simulink library "NeuroModelerLibrary"  (Simulink 10.2)
settings: Solver=ode45  StartTime=0.0  StopTime=10.0  RelTol=1e-3
libraries: $bdroot x672, simulink x5, neural x2
(part 1 of 5)
settings Model: Creator=Bakhshiev  LastModifiedBy=Bakhshiev

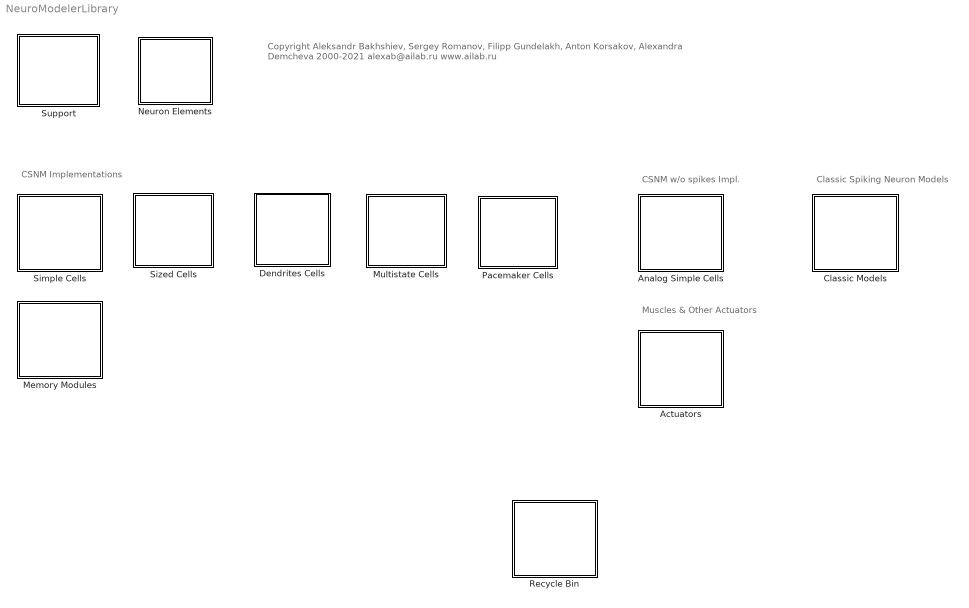
== system NeuroModelerLibrary ==
  note: CSNM Implementations
  note: Copyright Aleksandr Bakhshiev, Sergey Romanov, Filipp Gundelakh, Anton Korsakov, Alexandra Demcheva 2000-2021
      | alexab@ailab.ru
      | www.ailab.ru
  note: CSNM w/o spikes Impl.
  note: Muscles & Other Actuators
  note: Classic Spiking Neuron Models
  Actuators : Subsystem
  Analog Simple Cells : Subsystem
  Classic Models : Subsystem
  Dendrites Cells : Subsystem
  Memory Modules : Subsystem
  Multistate Cells : Subsystem
  Neuron Elements : Subsystem
  Pacemaker Cells : Subsystem
  Recycle Bin : Subsystem
  Simple Cells : Subsystem
  Sized Cells : Subsystem
  Support : Subsystem

== system NeuroModelerLibrary/Actuators ==
  Eye Muscle : Subsystem

== system NeuroModelerLibrary/Analog Simple Cells ==
  note: CSNM: version 0.2
  Simple Analog Neuron : Subsystem
  Simple Analog Neuron with PI : Subsystem  AncestorBlock=NeuroModelerLibrary/Analog Simple Cells/Simple Analog Neuron
  "Simple Tanh Analog Neuron " : Subsystem

== system NeuroModelerLibrary/Classic Models ==
  note: Neuron Models
  note: Synapse Models
  Alpha-Function Synapse (nonsmooth) : Subsystem  mask{tau_syn=2e-3, I_syn=1e-12, weight=1, delay=1e-3}
      mask prompts: tau_syn "Rise time of the exciatory synaptic alpha function"; I_syn "Synaptic current amplitude"
  Alpha-Function Synapse (smooth) : Subsystem  mask{tau_syn=2e-3, I_syn=1e-12, weight=1, delay=1e-3}
      mask prompts: tau_syn "Rise time of excitatory synaptic alpha function"; I_syn "Synaptic current amplitude"
  IaF Neuron : Subsystem  mask{tau_m=0.01, Cm=250e-12, I_const=0, E_L=-0.070, V_reset=-0.10, V_th=-0.055}
      mask prompts: tau_m "Membrane time constatnt"; Cm "Membrane capacity"; I_const "Constant input current"; E_L "Resting membrane potential"; V_reset "Reset membrane potential"; V_th "Threshold potential"
  IaF Neuron with refractory : Subsystem  mask{tau_m=0.01, Cm=250e-12, I_const=376e-12, E_L=-0.070, V_reset=-0.070, V_th=-0.055, tau_ref=0.002}
      mask prompts: tau_m "Membrane time constatnt"; Cm "Membrane capacity"; I_const "Constant input current"; E_L "Resting membrane potential"; V_reset "Reset membrane potential"; V_th "Threshold potential"; tau_ref "Refractory period"
  Static Synapse : Subsystem  mask{tau_syn=2e-3, I_syn=1e-8, weight=1, delay=1e-3}
      mask prompts: tau_syn "Rise time of the excitatory synaptic alpha function"; I_syn "Synaptic current amplitude"

== system NeuroModelerLibrary/Dendrites Cells ==
  note: CSNM: version 0.2
  Branching Dendrites Cell : Subsystem
  Branching Dendrites Cell ModGen : Subsystem  AncestorBlock=NeuroModelerLibrary/Dendrites Cells/Branching Dendrites Cell
  Branching Dendrites Cell ModGenSyn : Subsystem  AncestorBlock=NeuroModelerLibrary/Dendrites Cells/Branching Dendrites Cell
  Long Dendite Cell : Subsystem
  Long Dendite Cell ModGen : Subsystem  AncestorBlock=NeuroModelerLibrary/Dendrites Cells/Long Dendite Cell
  Long Dendite Cell ModGen(FBC) : Subsystem  AncestorBlock=NeuroModelerLibrary/Dendrites Cells/Long Dendite Cell
  Long Dendite Cell ModGenSyn : Subsystem  AncestorBlock=NeuroModelerLibrary/Dendrites Cells/Long Dendite Cell

== system NeuroModelerLibrary/Memory Modules ==
  note: CSNM: version 0.2
  Time-Memory Element : Subsystem
  Time-Memory PI Element : Subsystem

== system NeuroModelerLibrary/Multistate Cells ==
  note: CSNM: version 0.2
  Multistate Membrane Cell : Subsystem

== system NeuroModelerLibrary/Neuron Elements ==
  note: CSNM: version 0.1 (2010)
  note: CSNM: version 0.2 (2015)
  note: CSNM: version 0.3 (2021)
  CSNM Compartment : Subsystem  mask{ACm=1e-9, ARm=1e7, ECm=1e-9, ERm=1e7, ARFm=1e7, ERFm=1e7, U0=-0.070, sign=-1}
      mask prompts: ACm "Arresting Membrane Capacity"; ARm "Arresting Membrane Resistance"; ECm "Excitatory Membrane Capacity"; ERm "Excitatory Membrane Resistance"; ARFm "Feedback Arresting Resistance"; ERFm "Feedback Excitatory Resistance"; U0 "Synaptic EMF"; sign "Synaptic Weight Sign"
  CSNM LTZone : Subsystem  mask(Ion pump){NM=1, FB=2, T=-0.055, switchOff=-0.1}
      mask prompts: NM "Number of Input Membranes"; FB "Feedback Coeff"; T "On Threshold"; switchOff "Off Threshold"
  CSNM Synapse : Subsystem  mask{SecretionTC=0.001, DecompositionTC=0.005, UseKsi=off, Rs=2e7, ksi=1, U0=-0.070, Weight=1, sign=off}
      mask prompts: SecretionTC "Mediator Secretion"; DecompositionTC "Mediator Decomposition"; UseKsi "Use Presynaptic Inhubition"; Rs "Synaptic Resistance"; U0 "Synaptic EMF"; Weight "Synaptic Weight"; sign "Synaptic Weight Sign"
  CSNM Synapse-D : Subsystem  mask{SecretionTC=0.001, DecompositionTC=0.005, UseKsi=off, Rs=2e7, ksi=1, U0=-0.070, Weight=1, sign=off}
      mask prompts: SecretionTC "Mediator Secretion"; DecompositionTC "Mediator Decomposition"; UseKsi "Use Presynaptic Inhubition"; Rs "Synaptic Resistance"; U0 "Synaptic EMF"; Weight "Synaptic Weight"; sign "Synaptic Weight Sign"
  ContLTZone : Subsystem
  IaF Compartment : Subsystem  mask{tau_m=0.01, Cm=250e-12, I_const=0, E_L=-0.070, V_reset=-0.10, V_th=-0.055}
      mask prompts: tau_m "Membrane time constatnt"; Cm "Membrane capacity"; I_const "Constant input current"; E_L "Resting membrane potential"; V_reset "Reset membrane potential"; V_th "Threshold potential"
  IaF LTZone : Subsystem  mask{tau_m=0.01, Cm=250e-12, I_const=0, E_L=-0.070, V_reset=-0.10, V_th=-0.055}
      mask prompts: tau_m "Membrane time constatnt"; Cm "Membrane capacity"; I_const "Constant input current"; E_L "Resting membrane potential"; V_reset "Reset membrane potential"; V_th "Threshold potential"
  Ion System : Subsystem
  Ion System v0.1 : Subsystem
  LTZone : Subsystem  mask(Ion pump){NM=1, FB=1.7, IT=0.005, T=0.001}
      mask prompts: NM "Number of Input Membranes"; FB "Feedback Coeff"; IT "Input Time Constant"; T "Threshold"
  LTZone v0.1 : Subsystem  mask(Ion pump){Rc=1, Cc=0.001, RR=1, IT=0.005, T=10}
      mask prompts: Rc "Channel resistance"; Cc "Channel capacity"; RR "Recharge Resistance"; IT "Input TC"; T "Threshold"
  LTZoneV2 : Subsystem  mask(Ion pump){NM=1, FB=2, IT=0.001, T=-0.055, inertia=on, switchOff=-0.1}
      mask prompts: NM "Number of Input Membranes"; FB "Feedback Coeff"; IT "Input Time Constant"; T "Threshold"; inertia "Use inertia link"; switchOff "Switch off point"
  Multistate Membrane : Subsystem
  Neuro Membrane v0.1 : Subsystem  mask{ACm=0.1, ARm=0.1, ECm=0.01, ERm=0.1}
      mask prompts: ACm "Arresting Membrane Capacity"; ARm "Arresting Membrane Resistance"; ECm "Excitatory Membrane Capacity"; ERm "Excitatory Membrane Resistance"
  Simple Membrane : Subsystem  mask{ACm=1e-9, ARm=1e7, ECm=1e-9, ERm=1e7, ARFm=1e8, ERFm=1e8}
      mask prompts: ACm "Arresting Membrane Capacity"; ARm "Arresting Membrane Resistance"; ECm "Excitatory Membrane Capacity"; ERm "Excitatory Membrane Resistance"; ARFm "Feedback Arresting Resistance"; ERFm "Feedback Excitatory Resistance"
  Simple Synapse : $bdroot/Neuron Elements/Synapse  SecretionTC=0.001  DecompositionTC=0.01  UseKsi=off  ksi=2  gamma=1e8
  Synapse : Subsystem  mask{SecretionTC=0.001, DecompositionTC=0.01, UseKsi=on, ksi=2, gamma=1e8}
      mask prompts: SecretionTC "Mediator Secretion"; DecompositionTC "Mediator Decomposition"; UseKsi "Use Presynaptic Inhubition"
  Synapse Ion System v0.1 : Subsystem
  Synapse Membrane v0.1 : Subsystem  mask{ACm=0.1, ARm=0.1, ECm=0.01, ERm=0.1}
      mask prompts: ACm "Arresting Membrane Capacity"; ARm "Arresting Membrane Resistance"; ECm "Excitatory Membrane Capacity"; ERm "Excitatory Membrane Resistance"
  Synapse PresynInh v0.1 : $bdroot/Neuron Elements/Synapse v0.1  SecretionTC=0.001  DecompositionTC=0.1  ksi=2  gamma=1
  Synapse v0.1 : Subsystem  mask{SecretionTC=0.001, DecompositionTC=0.1, ksi=1, gamma=1}
      mask prompts: SecretionTC "Mediator Secretion"; DecompositionTC "Mediator Decomposition"

== system NeuroModelerLibrary/Pacemaker Cells ==
  note: CSNM: version 0.2
  Pacemaker1-1 Cell : Subsystem
  Pacemaker1-2 Cell : Subsystem
  Pacemaker1-3 Cell : Subsystem
  Pacemaker1-4 Cell : Subsystem
  Pacemaker2 Cell : Subsystem
  Pacemaker3 Cell : Subsystem
  Pacemaker4 Cell : Subsystem
  Pacemaker4x4 Cell : Subsystem
  Slow Pacemaker Cell : Subsystem

== system NeuroModelerLibrary/Recycle Bin ==
  note: Neural Networks Samples
  note: Neuron Samples
  note: Neuron Parts Samples
  Dendrite Neuron  Samples : Subsystem
  Membrane Samples : Subsystem
  Multistate Neuron  Samples : Subsystem
  PCN1 : Subsystem
  PCN2 : Subsystem
  Pacemaker Samples : Subsystem
  RCN : Subsystem
  Simple  Neural Networks : Subsystem
  Simple Neuron Samples : Subsystem
  Size Neuron  Samples : Subsystem
  Synapse Samples : Subsystem
  TCN : Subsystem

== system NeuroModelerLibrary/Simple Cells ==
  note: CSNM: version 0.2
  note: CSNM: version 0.1
  Afferent1 : Subsystem  mask{ExpCoeff=0.001, IncCoeff=0.999}
      mask prompts: ExpCoeff "Input Exp Coeff"; IncCoeff "Input Inc Coeff"
      mask DialogControl AffParams Prompt: Afferent Parameters
  Electric Simple Cell : Subsystem
  Electric Simple2 Cell : Subsystem
  Large  NewNeuron v0.1 : Subsystem
  Large PresynInh  NewNeuron v0.1 : Subsystem  AncestorBlock="NeuroModelerLibrary/Simple Cells/Large  NewNeuron v0.1"
  Simple Cell : Subsystem
  Simple Cell - Inertial : Subsystem  AncestorBlock=NeuroModelerLibrary/Simple Cells/Simple Cell
  Simple Cell MembraneCap : Subsystem
  Simple Cell MembraneCap[2] : Subsystem
  Small  NewNeuron v0.1 : Subsystem
  Small PresynInh NewNeuron v0.1 : Subsystem  AncestorBlock="NeuroModelerLibrary/Simple Cells/Small  NewNeuron v0.1"

== system NeuroModelerLibrary/Sized Cells ==
  note: CSNM: version 0.2
  note: CSNM: version 0.3
  note: Segmented IaF
  CSNM1x0 : Subsystem
  CSNM1x1 : Subsystem
  CSNM1x2 : Subsystem
  CSNM1x3 : Subsystem
  CSNM1x4-Syn4 : Subsystem
  CSNM2x0 : Subsystem
  CSNM2x1 : Subsystem
  CSNM2x2 : Subsystem
  CSNM2x3 : Subsystem
  CSNM3x0 : Subsystem
  CSNM3x1 : Subsystem
  CSNM3x2 : Subsystem
  CSNM3x3 : Subsystem
  CSNM4x0 : Subsystem
  CSNM4x1 : Subsystem
  CSNM4x2 : Subsystem
  CSNM4x3 : Subsystem
  Cell IaF 1x4 : Subsystem
  Cell IaF 1x4-Syn4 : Subsystem
  Cell IaF 2x4 : Subsystem
  Cell IaF 3x4 : Subsystem
  Cell IaF 4x4 : Subsystem
  Size Cell : Subsystem
  Size2 Cell : Subsystem
  Size3 Cell : Subsystem
  Size3 Cell ModSynS1A1 : Subsystem
  Size4 Cell : Subsystem
  Size6 Cell : Subsystem

== system NeuroModelerLibrary/Support ==
  Electric Engine Model : Subsystem
  Inertial Link : Subsystem
  Inertial Link With Reset : Subsystem
  Sign Separator : Subsystem
  Two-output Pulse Generator : Subsystem  mask{A=1, P1=200, P2=200, PW=1, ST=0.001, OOn1=0.5, OOff1=0.6, OOn2=1.1, OOff2=1.2}
      mask prompts: A "Amplitude"; P1 "Out1: Period (number of samples)"; P2 "Out2: Period (number of samples)"; PW "Pulse Width (number of samples)"; ST "Sample Time"; OOn1 "Out1 On (seconds)"; OOff1 "Out1 Off (seconds)"; OOn2 "Out2 On (seconds)"; OOff2 "Out2 Off (seconds)"

== system NeuroModelerLibrary/Actuators/Eye Muscle ==
  In1 : Inport
  Gain : Gain  Gain=380
  Gain1 : Gain  Gain=0.75
  Gain2 : Gain  Gain=195
  Gain3 : Gain  Gain=0.75
  Gain4 : Gain  Gain=30
  Gain5 : Gain  Gain=0.45
  Integrator : Integrator
  Integrator1 : Integrator
  Integrator2 : Integrator
  Subtract : Sum  Inputs=+--
  Subtract1 : Sum  Inputs=+-
  Out1 : Outport
  wires:
  In1/1 -> Subtract/1
  Subtract/1 -> Gain/1
  Gain1/1 -> Subtract/3
  Integrator/1 -> Gain1/1, Subtract1/1
  Integrator1/1 -> Gain4/1, Gain3/1
  Gain2/1 -> Integrator1/1
  Gain4/1 -> Integrator2/1
  Subtract1/1 -> Gain2/1
  Gain/1 -> Integrator/1
  Integrator2/1 -> Out1/1, Gain5/1
  Gain3/1 -> Subtract1/2
  Gain5/1 -> Subtract/2

== system NeuroModelerLibrary/Analog Simple Cells/Simple Analog Neuron ==
  Ex Input 1 : Inport
  Ex Input 2 : Inport  Port=2
  Ar Input 2 : Inport  Port=3
  Ar Input 1 : Inport  Port=4
  C2 : Constant
  C3 : Constant  Value=-1
  ContLTZone1 : $bdroot/Neuron Elements/ContLTZone  SystemSampleTime=-1  VariantActivationTime=update diagram  Latency=0  AutoFrameSizeCalculation=off
  Simple Membrane1 : $bdroot/Neuron Elements/Simple Membrane  ACm=1e-9  ARm=1e7  ECm=1e-9  ERm=1e7  ARFm=1e8  ERFm=1e8
  Simple Synapse{,1..3} (4 alike) : $bdroot/Neuron Elements/Synapse  SecretionTC=0.001  DecompositionTC=0.01  UseKsi=off  ksi=2  gamma=1e8
  Sum4 : Sum  InputSameDT=on  SaturateOnIntegerOverflow=on  OutDataTypeStr=Inherit: Same as first input
  Sum7 : Sum  InputSameDT=on  SaturateOnIntegerOverflow=on  OutDataTypeStr=Inherit: Same as first input
  Sum8 : Sum  InputSameDT=on  SaturateOnIntegerOverflow=on  OutDataTypeStr=Inherit: Same as first input
  Out : Outport  VectorParamsAs1DForOutWhenUnconnected=off
  Potential : Outport  Port=2  VectorParamsAs1DForOutWhenUnconnected=off
  wires:
  Ex Input 2/1 -> Simple Synapse1/1
  ContLTZone1/1 -> Out/1
  Simple Synapse3/1 -> Sum8/2
  Simple Synapse2/1 -> Sum8/1
  Sum8/1 -> Simple Membrane1/5
  Ar Input 2/1 -> Simple Synapse3/1
  Simple Synapse1/1 -> Sum4/2
  Simple Synapse/1 -> Sum4/1
  Sum4/1 -> Simple Membrane1/1
  Ar Input 1/1 -> Simple Synapse2/1
  Ex Input 1/1 -> Simple Synapse/1
  Sum7/1 -> ContLTZone1/1, Potential/1
  Simple Membrane1/2 -> Sum7/2
  Simple Membrane1/1 -> Sum7/1
  C3/1 -> Simple Membrane1/4
  C2/1 -> Simple Membrane1/2

== system NeuroModelerLibrary/Analog Simple Cells/Simple Analog Neuron with PI ==
  Ex Input 1 : Inport
  Ex Input 2 : Inport  Port=2
  Ar Input 2 : Inport  Port=3
  Ar Input 1 : Inport  Port=4
  C2 : Constant
  C3 : Constant  Value=-1
  ContLTZone1 : $bdroot/Neuron Elements/ContLTZone  SystemSampleTime=-1  VariantActivationTime=update diagram  Latency=0  AutoFrameSizeCalculation=off
  Simple Membrane1 : $bdroot/Neuron Elements/Simple Membrane  ACm=1e-9  ARm=1e7  ECm=1e-9  ERm=1e7  ARFm=1e8  ERFm=1e8
  Simple Synapse{,1..3} (4 alike) : $bdroot/Neuron Elements/Synapse  SecretionTC=0.001  DecompositionTC=0.01  UseKsi=on  ksi=2  gamma=1e8
  Sum4 : Sum  InputSameDT=on  SaturateOnIntegerOverflow=on  OutDataTypeStr=Inherit: Same as first input
  Sum7 : Sum  InputSameDT=on  SaturateOnIntegerOverflow=on  OutDataTypeStr=Inherit: Same as first input
  Sum8 : Sum  InputSameDT=on  SaturateOnIntegerOverflow=on  OutDataTypeStr=Inherit: Same as first input
  Out : Outport  VectorParamsAs1DForOutWhenUnconnected=off
  Potential : Outport  Port=2  VectorParamsAs1DForOutWhenUnconnected=off
  wires:
  Ex Input 2/1 -> Simple Synapse1/1
  ContLTZone1/1 -> Out/1
  Simple Synapse3/1 -> Sum8/2
  Simple Synapse2/1 -> Sum8/1
  Sum8/1 -> Simple Membrane1/5
  Ar Input 2/1 -> Simple Synapse3/1
  Simple Synapse1/1 -> Sum4/2
  Simple Synapse/1 -> Sum4/1
  Sum4/1 -> Simple Membrane1/1
  Ar Input 1/1 -> Simple Synapse2/1
  Ex Input 1/1 -> Simple Synapse/1
  Sum7/1 -> ContLTZone1/1, Potential/1
  Simple Membrane1/2 -> Sum7/2
  Simple Membrane1/1 -> Sum7/1
  C3/1 -> Simple Membrane1/4
  C2/1 -> Simple Membrane1/2

== system NeuroModelerLibrary/Analog Simple Cells/Simple Tanh Analog Neuron  ==
  Ex Input 1 : Inport
  Ex Input 2 : Inport  Port=2
  Ar Input 2 : Inport  Port=3
  Ar Input 1 : Inport  Port=4
  C2 : Constant
  C3 : Constant  Value=-1
  Simple Membrane1 : $bdroot/Neuron Elements/Simple Membrane  ACm=1e-9  ARm=1e7  ECm=1e-9  ERm=1e7  ARFm=1e8  ERFm=1e8
  Simple Synapse{,1..3} (4 alike) : $bdroot/Neuron Elements/Simple Synapse  SecretionTC=0.001  DecompositionTC=0.01  gamma=1e8
  Sum4 : Sum  InputSameDT=on  SaturateOnIntegerOverflow=on  OutDataTypeStr=Inherit: Same as first input
  Sum7 : Sum  InputSameDT=on  SaturateOnIntegerOverflow=on  OutDataTypeStr=Inherit: Same as first input
  Sum8 : Sum  InputSameDT=on  SaturateOnIntegerOverflow=on  OutDataTypeStr=Inherit: Same as first input
  tansig : neural/Transfer Functions/tansig
  Out : Outport  VectorParamsAs1DForOutWhenUnconnected=off
  Potential : Outport  Port=2  VectorParamsAs1DForOutWhenUnconnected=off
  wires:
  C2/1 -> Simple Membrane1/2
  C3/1 -> Simple Membrane1/4
  Simple Membrane1/1 -> Sum7/1
  Simple Membrane1/2 -> Sum7/2
  Sum7/1 -> tansig/1, Potential/1
  Ex Input 1/1 -> Simple Synapse/1
  Ar Input 1/1 -> Simple Synapse2/1
  Sum4/1 -> Simple Membrane1/1
  Simple Synapse/1 -> Sum4/1
  Simple Synapse1/1 -> Sum4/2
  Ar Input 2/1 -> Simple Synapse3/1
  Sum8/1 -> Simple Membrane1/5
  Simple Synapse2/1 -> Sum8/1
  Simple Synapse3/1 -> Sum8/2
  tansig/1 -> Out/1
  Ex Input 2/1 -> Simple Synapse1/1

== system NeuroModelerLibrary/Classic Models/Alpha-Function Synapse (nonsmooth) ==
  pulse input : Inport
  -1/tau_syn : Gain  Gain=-1/(tau_syn)
  Clock : Clock
  Constant : Constant
  Constant1 : Constant  Value=0
  Constant2 : Constant  Value=0
  Delay : TransportDelay  DelayTime=delay
  I_syn : Gain  Gain=I_syn
  Math Function : Math  SaturateOnIntegerOverflow=on
  MinMax Running Resettable : simulink/Math Operations/MinMax Running Resettable  Function=max  vinit=0.0
  Product1 : Product
  Sum : Sum  Inputs=-+|
  Switch : Switch  Criteria=u2 > Threshold
  Switch1 : Switch  Criteria=u2 > Threshold
  Triggered Subsystem : Subsystem  TreatAsAtomicUnit=on
  Weight : Gain  Gain=weight
  i_syn : Outport
  wires:
  Delay/1 -> i_syn/1
  Switch1/1 -> Weight/1
  MinMax Running Resettable/1 -> Switch1/2
  Product1/1 -> Switch1/1
  Constant2/1 -> Switch1/3
  Constant/1 -> Switch/1
  Constant1/1 -> Switch/3
  Triggered Subsystem/1(Out1) -> Sum/1
  pulse input/1 -> MinMax Running Resettable/1, Triggered Subsystem/Trigger
  Clock/1 -> Triggered Subsystem/1(In1), Sum/2
  Switch/1 -> Product1/2
  Math Function/1 -> I_syn/1
  -1/tau_syn/1 -> Math Function/1
  Sum/1 -> Switch/2, -1/tau_syn/1
  Weight/1 -> Delay/1
  I_syn/1 -> Product1/1

== system NeuroModelerLibrary/Classic Models/Alpha-Function Synapse (smooth) ==
  pulse input : Inport
  -1/tau_syn : Gain  Gain=-1/(tau_syn)
  1/tau_syn : Gain  Gain=1/(tau_syn)
  Clock : Clock
  Constant : Constant
  Constant1 : Constant  Value=0
  Constant2 : Constant  Value=0
  Delay : TransportDelay  DelayTime=delay
  Gain4 : Gain  Gain=exp(1)
  I_syn : Gain  Gain=I_syn
  Math Function : Math  SaturateOnIntegerOverflow=on
  MinMax Running Resettable : simulink/Math Operations/MinMax Running Resettable  Function=max  vinit=0.0
  Product : Product
  Product1 : Product
  Sum : Sum  Inputs=-+|
  Switch : Switch  Criteria=u2 > Threshold
  Switch1 : Switch  Criteria=u2 > Threshold
  Triggered Subsystem : Subsystem  TreatAsAtomicUnit=on
  Weight : Gain  Gain=weight
  i_syn : Outport
  wires:
  Delay/1 -> i_syn/1
  Switch1/1 -> Weight/1
  MinMax Running Resettable/1 -> Switch1/2
  Product1/1 -> Switch1/1
  Constant2/1 -> Switch1/3
  Product/1 -> I_syn/1
  Constant/1 -> Switch/1
  Constant1/1 -> Switch/3
  Triggered Subsystem/1(Out1) -> Sum/1
  pulse input/1 -> MinMax Running Resettable/1, Triggered Subsystem/Trigger
  Clock/1 -> Triggered Subsystem/1(In1), Sum/2
  Switch/1 -> Product1/2
  Math Function/1 -> Product/2
  -1/tau_syn/1 -> Math Function/1
  Gain4/1 -> 1/tau_syn/1
  Sum/1 -> Gain4/1, -1/tau_syn/1, Switch/2
  Weight/1 -> Delay/1
  1/tau_syn/1 -> Product/1
  I_syn/1 -> Product1/1

== system NeuroModelerLibrary/Classic Models/IaF Neuron ==
  i_syn : Inport
  Constant1 : Constant  Value=V_reset
  Constant10 : Constant  Value=tau_m
  Constant11 : Constant  Value=E_L
  Constant12 : Constant  Value=I_const
  Constant2 : Constant
  Constant6 : Constant  Value=0
  Gain1 : Gain
  Gain2 : Gain  Gain=tau_m/Cm
  Gain3 : Gain  Gain=tau_m/Cm
  Inertial Link With Reset : $bdroot/Support/Inertial Link With Reset  SystemSampleTime=-1  VariantActivationTime=update diagram  Latency=0  AutoFrameSizeCalculation=off
  S1 : Switch  Threshold=V_th  SaturateOnIntegerOverflow=on  InputSameDT=on
  S3 : Switch  Threshold=V_th  SaturateOnIntegerOverflow=on  InputSameDT=on
  Sum1 : Sum
  Sum3 : Sum
  Vm : Outport
  wires:
  S3/1 -> Vm/1
  i_syn/1 -> Gain3/1
  S1/1 -> Inertial Link With Reset/4
  Constant1/1 -> Inertial Link With Reset/3, S3/1
  Inertial Link With Reset/1 -> S3/2, S3/3, S1/2
  Gain1/1 -> Inertial Link With Reset/1
  Sum3/1 -> Gain1/1
  Constant6/1 -> S1/3
  Constant2/1 -> S1/1
  Gain2/1 -> Sum1/2
  Sum1/1 -> Sum3/1
  Gain3/1 -> Sum1/1
  Constant10/1 -> Inertial Link With Reset/2
  Constant11/1 -> Sum3/2
  Constant12/1 -> Gain2/1

== system NeuroModelerLibrary/Classic Models/IaF Neuron with refractory ==
  i_syn : Inport
  Clock : Clock
  Constant1 : Constant  Value=V_reset
  Constant10 : Constant  Value=tau_m
  Constant11 : Constant  Value=E_L
  Constant12 : Constant  Value=I_const
  Constant2 : Constant
  Constant3 : Constant  Value=E_L
  Constant4 : Constant
  Constant5 : Constant  Value=0
  Constant6 : Constant  Value=0
  Gain3 : Gain  Gain=tau_m/Cm
  Inertial Link With Reset1 : $bdroot/Support/Inertial Link With Reset  SystemSampleTime=-1  VariantActivationTime=update diagram  Latency=0  AutoFrameSizeCalculation=off
  S1 : Switch  Threshold=V_th  SaturateOnIntegerOverflow=on  InputSameDT=on
  S2 : Switch  Threshold=tau_ref  SaturateOnIntegerOverflow=on  InputSameDT=on
  S3 : Switch  Threshold=V_th  SaturateOnIntegerOverflow=on  InputSameDT=on
  S4 : Switch  Threshold=V_th - 0.000005  SaturateOnIntegerOverflow=on  InputSameDT=on
  Sum : Sum  Inputs=-+|
  Sum1 : Sum
  Sum3 : Sum
  Triggered Subsystem : Subsystem  TreatAsAtomicUnit=on
  Vm : Outport
  wires:
  S4/1 -> Triggered Subsystem/Trigger
  Constant5/1 -> S4/3
  Inertial Link With Reset1/1 -> S1/2, S3/2, S3/3, S4/2
  Constant4/1 -> S4/1
  Constant3/1 -> S2/3
  S2/1 -> Vm/1
  Sum/1 -> S2/2
  Clock/1 -> Triggered Subsystem/1(In1), Sum/2
  Triggered Subsystem/1(Out1) -> Sum/1
  Gain3/1 -> Sum3/1  "Input"
  S3/1 -> S2/1
  S1/1 -> Inertial Link With Reset1/4
  Constant1/1 -> Inertial Link With Reset1/3, S3/1
  Sum3/1 -> Inertial Link With Reset1/1  "Value"
  Constant6/1 -> S1/3
  Constant2/1 -> S1/1
  Constant12/1 -> Sum1/2
  Sum1/1 -> Gain3/1
  i_syn/1 -> Sum1/1
  Constant10/1 -> Inertial Link With Reset1/2
  Constant11/1 -> Sum3/2

== system NeuroModelerLibrary/Classic Models/Static Synapse ==
  pulse input : Inport
  Gain : Gain  Gain=weight
  Gain6 : Gain  Gain=I_syn
  Transfer Fcn : TransferFcn  Denominator="[(tau_syn*tau_syn)  (2*tau_syn)  1]"
  Transport Delay : TransportDelay  DelayTime=delay
  i_syn : Outport
  wires:
  pulse input/1 -> Transfer Fcn/1
  Transfer Fcn/1 -> Gain6/1
  Gain6/1 -> Gain/1
  Gain/1 -> Transport Delay/1
  Transport Delay/1 -> i_syn/1

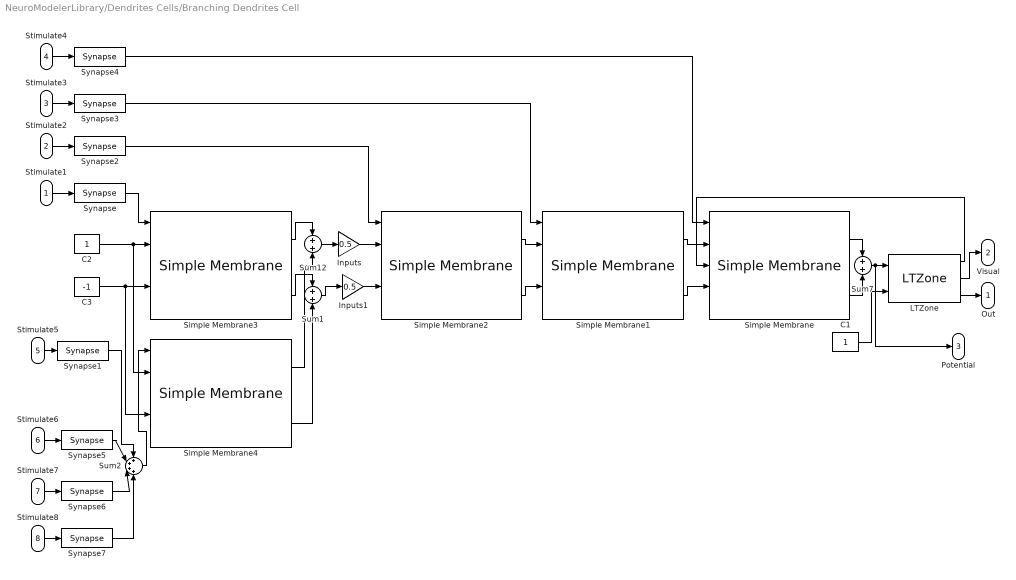
== system NeuroModelerLibrary/Dendrites Cells/Branching Dendrites Cell ==
  Stimulate1 : Inport
  Stimulate2 : Inport  Port=2
  Stimulate3 : Inport  Port=3
  Stimulate4 : Inport  Port=4
  Stimulate5 : Inport  Port=5
  Stimulate6 : Inport  Port=6
  Stimulate7 : Inport  Port=7
  Stimulate8 : Inport  Port=8
  C1 : Constant
  C2 : Constant
  C3 : Constant  Value=-1
  Inputs : Gain  Gain=0.5  OutDataTypeStr=Inherit: Same as input  ParamDataTypeStr=Inherit: Same as input
  Inputs1 : Gain  Gain=0.5  OutDataTypeStr=Inherit: Same as input  ParamDataTypeStr=Inherit: Same as input
  LTZone : $bdroot/Neuron Elements/LTZone  NM=1  FB=1.7  IT=0.005  T=0.001
  Simple Membrane{,1..4} (5 alike) : $bdroot/Neuron Elements/Simple Membrane  ACm=1e-9  ARm=1e7  ECm=1e-9  ERm=1e7  ARFm=1e8  ERFm=1e8
  Sum1 : Sum  InputSameDT=on  SaturateOnIntegerOverflow=on  OutDataTypeStr=Inherit: Same as first input
  Sum12 : Sum  InputSameDT=on  SaturateOnIntegerOverflow=on  OutDataTypeStr=Inherit: Same as first input
  Sum2 : Sum  Inputs=++++  InputSameDT=on  SaturateOnIntegerOverflow=on  OutDataTypeStr=Inherit: Same as first input
  Sum7 : Sum  InputSameDT=on  SaturateOnIntegerOverflow=on  OutDataTypeStr=Inherit: Same as first input
  Synapse{,1..7} (8 alike) : $bdroot/Neuron Elements/Synapse  SecretionTC=0.001  DecompositionTC=0.01  UseKsi=on  ksi=2  gamma=1e8
  Out : Outport  VectorParamsAs1DForOutWhenUnconnected=off
  Visual : Outport  Port=2  VectorParamsAs1DForOutWhenUnconnected=off
  Potential : Outport  Port=3  VectorParamsAs1DForOutWhenUnconnected=off
  wires:
  Synapse7/1 -> Sum2/4
  Stimulate8/1 -> Synapse7/1
  Synapse6/1 -> Sum2/3
  Stimulate7/1 -> Synapse6/1
  Stimulate6/1 -> Synapse5/1
  Stimulate4/1 -> Synapse4/1
  Synapse4/1 -> Simple Membrane/1
  Stimulate3/1 -> Synapse3/1
  Synapse3/1 -> Simple Membrane1/1
  Stimulate2/1 -> Synapse2/1
  Synapse2/1 -> Simple Membrane2/1
  Synapse/1 -> Simple Membrane3/1
  C2/1 -> Simple Membrane4/2, Simple Membrane3/2
  C3/1 -> Simple Membrane4/4, Simple Membrane3/4
  LTZone/2 -> Visual/1
  LTZone/3 -> Out/1
  C1/1 -> LTZone/2
  Stimulate1/1 -> Synapse/1
  Stimulate5/1 -> Synapse1/1
  Simple Membrane1/1 -> Simple Membrane/2
  Simple Membrane1/2 -> Simple Membrane/4
  Sum7/1 -> Potential/1, LTZone/1
  LTZone/1 -> Simple Membrane/3
  Simple Membrane/1 -> Sum7/1
  Simple Membrane/2 -> Sum7/2
  Simple Membrane4/2 -> Sum1/2
  Simple Membrane4/1 -> Sum12/2
  Sum12/1 -> Inputs/1
  Sum1/1 -> Inputs1/1
  Simple Membrane3/2 -> Sum1/1
  Simple Membrane3/1 -> Sum12/1
  Simple Membrane2/1 -> Simple Membrane1/2
  Simple Membrane2/2 -> Simple Membrane1/4
  Sum2/1 -> Simple Membrane4/1
  Synapse1/1 -> Sum2/1
  Inputs/1 -> Simple Membrane2/2
  Inputs1/1 -> Simple Membrane2/4
  Synapse5/1 -> Sum2/2

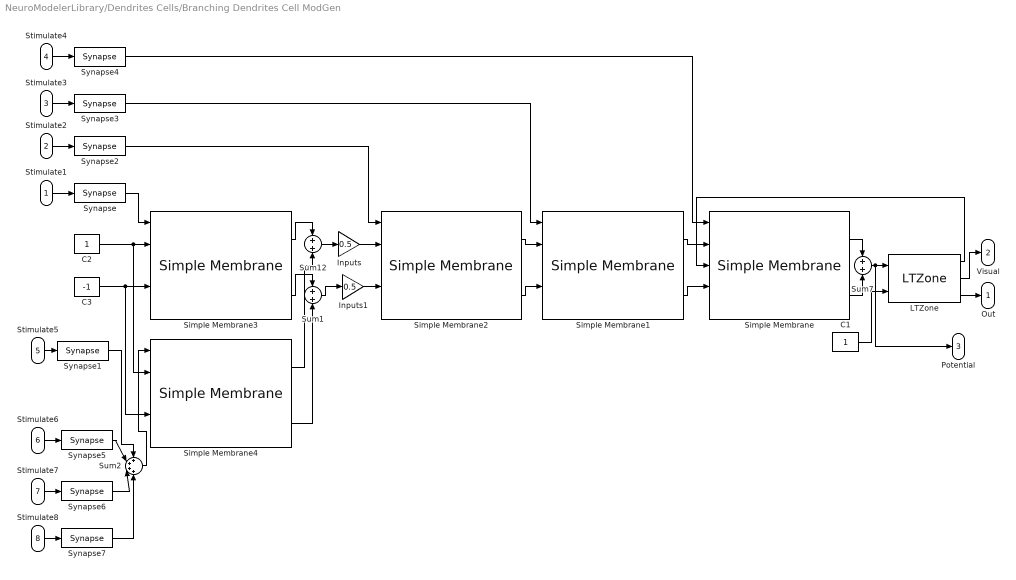
== system NeuroModelerLibrary/Dendrites Cells/Branching Dendrites Cell ModGen ==
  Stimulate1 : Inport
  Stimulate2 : Inport  Port=2
  Stimulate3 : Inport  Port=3
  Stimulate4 : Inport  Port=4
  Stimulate5 : Inport  Port=5
  Stimulate6 : Inport  Port=6
  Stimulate7 : Inport  Port=7
  Stimulate8 : Inport  Port=8
  C1 : Constant
  C2 : Constant
  C3 : Constant  Value=-1
  Inputs : Gain  Gain=0.5  OutDataTypeStr=Inherit: Same as input  ParamDataTypeStr=Inherit: Same as input
  Inputs1 : Gain  Gain=0.5  OutDataTypeStr=Inherit: Same as input  ParamDataTypeStr=Inherit: Same as input
  LTZone : $bdroot/Neuron Elements/LTZone  NM=1  FB=1.7  IT=0.005  T=0.1
  Simple Membrane{,1..4} (5 alike) : $bdroot/Neuron Elements/Simple Membrane  ACm=1e-9  ARm=1e7  ECm=1e-9  ERm=1e7  ARFm=1e8  ERFm=1e8
  Sum1 : Sum  InputSameDT=on  SaturateOnIntegerOverflow=on  OutDataTypeStr=Inherit: Same as first input
  Sum12 : Sum  InputSameDT=on  SaturateOnIntegerOverflow=on  OutDataTypeStr=Inherit: Same as first input
  Sum2 : Sum  Inputs=++++  InputSameDT=on  SaturateOnIntegerOverflow=on  OutDataTypeStr=Inherit: Same as first input
  Sum7 : Sum  InputSameDT=on  SaturateOnIntegerOverflow=on  OutDataTypeStr=Inherit: Same as first input
  Synapse{,1..7} (8 alike) : $bdroot/Neuron Elements/Synapse  SecretionTC=0.001  DecompositionTC=0.01  UseKsi=on  ksi=2  gamma=1e8
  Out : Outport  VectorParamsAs1DForOutWhenUnconnected=off
  Visual : Outport  Port=2  VectorParamsAs1DForOutWhenUnconnected=off
  Potential : Outport  Port=3  VectorParamsAs1DForOutWhenUnconnected=off
  wires:
  Synapse5/1 -> Sum2/2
  Inputs1/1 -> Simple Membrane2/4
  Inputs/1 -> Simple Membrane2/2
  Synapse1/1 -> Sum2/1
  Sum2/1 -> Simple Membrane4/1
  Simple Membrane2/2 -> Simple Membrane1/4
  Simple Membrane2/1 -> Simple Membrane1/2
  Simple Membrane3/1 -> Sum12/1
  Simple Membrane3/2 -> Sum1/1
  Sum1/1 -> Inputs1/1
  Sum12/1 -> Inputs/1
  Simple Membrane4/1 -> Sum12/2
  Simple Membrane4/2 -> Sum1/2
  Simple Membrane/2 -> Sum7/2
  Simple Membrane/1 -> Sum7/1
  LTZone/1 -> Simple Membrane/3
  Sum7/1 -> LTZone/1, Potential/1
  Simple Membrane1/2 -> Simple Membrane/4
  Simple Membrane1/1 -> Simple Membrane/2
  Stimulate5/1 -> Synapse1/1
  Stimulate1/1 -> Synapse/1
  C1/1 -> LTZone/2
  LTZone/3 -> Out/1
  LTZone/2 -> Visual/1
  C3/1 -> Simple Membrane3/4, Simple Membrane4/4
  C2/1 -> Simple Membrane3/2, Simple Membrane4/2
  Synapse/1 -> Simple Membrane3/1
  Synapse2/1 -> Simple Membrane2/1
  Stimulate2/1 -> Synapse2/1
  Synapse3/1 -> Simple Membrane1/1
  Stimulate3/1 -> Synapse3/1
  Synapse4/1 -> Simple Membrane/1
  Stimulate4/1 -> Synapse4/1
  Stimulate6/1 -> Synapse5/1
  Stimulate7/1 -> Synapse6/1
  Synapse6/1 -> Sum2/3
  Stimulate8/1 -> Synapse7/1
  Synapse7/1 -> Sum2/4

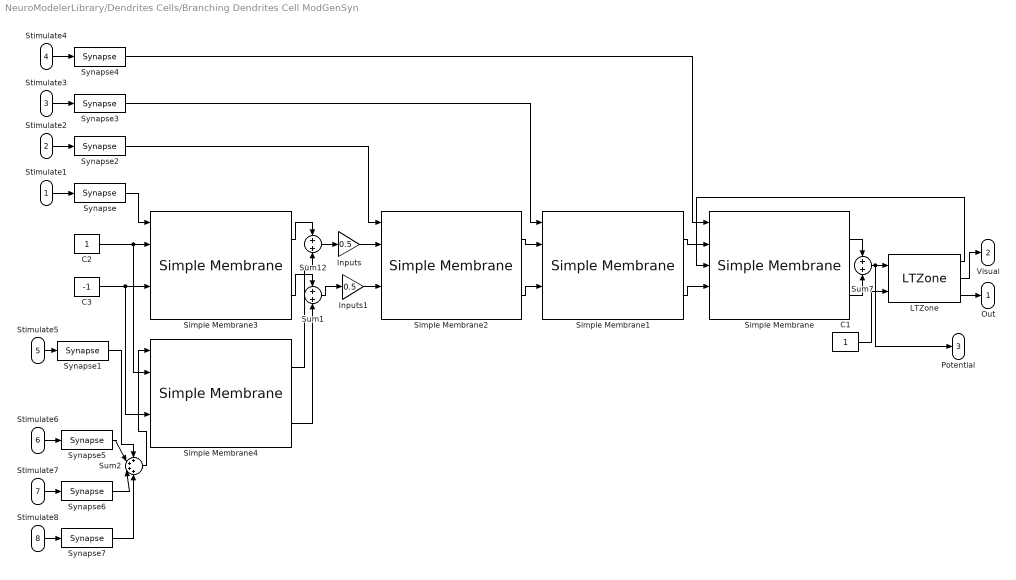
== system NeuroModelerLibrary/Dendrites Cells/Branching Dendrites Cell ModGenSyn ==
  Stimulate1 : Inport
  Stimulate2 : Inport  Port=2
  Stimulate3 : Inport  Port=3
  Stimulate4 : Inport  Port=4
  Stimulate5 : Inport  Port=5
  Stimulate6 : Inport  Port=6
  Stimulate7 : Inport  Port=7
  Stimulate8 : Inport  Port=8
  C1 : Constant
  C2 : Constant
  C3 : Constant  Value=-1
  Inputs : Gain  Gain=0.5  OutDataTypeStr=Inherit: Same as input  ParamDataTypeStr=Inherit: Same as input
  Inputs1 : Gain  Gain=0.5  OutDataTypeStr=Inherit: Same as input  ParamDataTypeStr=Inherit: Same as input
  LTZone : $bdroot/Neuron Elements/LTZone  NM=1  FB=2  IT=0.005  T=0.1
  Simple Membrane{,1..4} (5 alike) : $bdroot/Neuron Elements/Simple Membrane  ACm=1e-9  ARm=1e7  ECm=1e-9  ERm=1e7  ARFm=1e8  ERFm=1e8
  Sum1 : Sum  InputSameDT=on  SaturateOnIntegerOverflow=on  OutDataTypeStr=Inherit: Same as first input
  Sum12 : Sum  InputSameDT=on  SaturateOnIntegerOverflow=on  OutDataTypeStr=Inherit: Same as first input
  Sum2 : Sum  Inputs=++++  InputSameDT=on  SaturateOnIntegerOverflow=on  OutDataTypeStr=Inherit: Same as first input
  Sum7 : Sum  InputSameDT=on  SaturateOnIntegerOverflow=on  OutDataTypeStr=Inherit: Same as first input
  Synapse{,1..7} (8 alike) : $bdroot/Neuron Elements/Synapse  SecretionTC=0.001  DecompositionTC=0.01  UseKsi=on  ksi=1  gamma=1e8
  Out : Outport
  Visual : Outport  Port=2
  Potential : Outport  Port=3
  wires:
  Synapse7/1 -> Sum2/4
  Stimulate8/1 -> Synapse7/1
  Synapse6/1 -> Sum2/3
  Stimulate7/1 -> Synapse6/1
  Stimulate6/1 -> Synapse5/1
  Stimulate4/1 -> Synapse4/1
  Synapse4/1 -> Simple Membrane/1
  Stimulate3/1 -> Synapse3/1
  Synapse3/1 -> Simple Membrane1/1
  Stimulate2/1 -> Synapse2/1
  Synapse2/1 -> Simple Membrane2/1
  Synapse/1 -> Simple Membrane3/1
  C2/1 -> Simple Membrane4/2, Simple Membrane3/2
  C3/1 -> Simple Membrane4/4, Simple Membrane3/4
  LTZone/2 -> Visual/1
  LTZone/3 -> Out/1
  C1/1 -> LTZone/2
  Stimulate1/1 -> Synapse/1
  Stimulate5/1 -> Synapse1/1
  Simple Membrane1/1 -> Simple Membrane/2
  Simple Membrane1/2 -> Simple Membrane/4
  Sum7/1 -> Potential/1, LTZone/1
  LTZone/1 -> Simple Membrane/3
  Simple Membrane/1 -> Sum7/1
  Simple Membrane/2 -> Sum7/2
  Simple Membrane4/2 -> Sum1/2
  Simple Membrane4/1 -> Sum12/2
  Sum12/1 -> Inputs/1
  Sum1/1 -> Inputs1/1
  Simple Membrane3/2 -> Sum1/1
  Simple Membrane3/1 -> Sum12/1
  Simple Membrane2/1 -> Simple Membrane1/2
  Simple Membrane2/2 -> Simple Membrane1/4
  Sum2/1 -> Simple Membrane4/1
  Synapse1/1 -> Sum2/1
  Inputs/1 -> Simple Membrane2/2
  Inputs1/1 -> Simple Membrane2/4
  Synapse5/1 -> Sum2/2

== system NeuroModelerLibrary/Dendrites Cells/Long Dendite Cell ==
  Stimulate1 : Inport
  Stimulate2 : Inport  Port=2
  Stimulate3 : Inport  Port=3
  Stimulate4 : Inport  Port=4
  Arresting1 : Inport  Port=5
  Arresting2 : Inport  Port=6
  Arresting3 : Inport  Port=7
  Arresting4 : Inport  Port=8
  C1 : Constant
  C2 : Constant
  C3 : Constant  Value=-1
  LTZone : $bdroot/Neuron Elements/LTZone  NM=1  FB=1.7  IT=0.005  T=0.001
  Simple Membrane{,1..3} (4 alike) : $bdroot/Neuron Elements/Simple Membrane  ACm=1e-9  ARm=1e7  ECm=1e-9  ERm=1e7  ARFm=1e8  ERFm=1e8
  Sum12 : Sum  InputSameDT=on  SaturateOnIntegerOverflow=on  OutDataTypeStr=Inherit: Same as first input
  Sum7 : Sum  InputSameDT=on  SaturateOnIntegerOverflow=on  OutDataTypeStr=Inherit: Same as first input
  Synapse{,1..7} (8 alike) : $bdroot/Neuron Elements/Synapse  SecretionTC=0.001  DecompositionTC=0.01  UseKsi=on  ksi=2  gamma=1e8
  Out : Outport  VectorParamsAs1DForOutWhenUnconnected=off
  Visual : Outport  Port=2  VectorParamsAs1DForOutWhenUnconnected=off
  Potential : Outport  Port=3  VectorParamsAs1DForOutWhenUnconnected=off
  wires:
  Simple Membrane/2 -> Sum7/2
  Simple Membrane/1 -> Sum7/1
  LTZone/1 -> Simple Membrane/3
  Sum7/1 -> Potential/1, LTZone/1
  Simple Membrane1/2 -> Sum12/2, Simple Membrane/4
  Simple Membrane1/1 -> Sum12/1, Simple Membrane/2
  Arresting1/1 -> Synapse1/1
  Stimulate1/1 -> Synapse/1
  C1/1 -> LTZone/2
  LTZone/3 -> Out/1
  LTZone/2 -> Visual/1
  Simple Membrane2/1 -> Simple Membrane1/2
  Simple Membrane2/2 -> Simple Membrane1/4
  Simple Membrane3/1 -> Simple Membrane2/2
  Simple Membrane3/2 -> Simple Membrane2/4
  Synapse1/1 -> Simple Membrane3/5
  C3/1 -> Simple Membrane3/4
  C2/1 -> Simple Membrane3/2
  Synapse/1 -> Simple Membrane3/1
  Synapse2/1 -> Simple Membrane2/1
  Stimulate2/1 -> Synapse2/1
  Synapse3/1 -> Simple Membrane1/1
  Stimulate3/1 -> Synapse3/1
  Synapse4/1 -> Simple Membrane/1
  Stimulate4/1 -> Synapse4/1
  Arresting2/1 -> Synapse5/1
  Synapse5/1 -> Simple Membrane2/5
  Arresting3/1 -> Synapse6/1
  Synapse6/1 -> Simple Membrane1/5
  Arresting4/1 -> Synapse7/1
  Synapse7/1 -> Simple Membrane/5

== system NeuroModelerLibrary/Dendrites Cells/Long Dendite Cell ModGen ==
  Stimulate1 : Inport
  Stimulate2 : Inport  Port=2
  Stimulate3 : Inport  Port=3
  Stimulate4 : Inport  Port=4
  Arresting1 : Inport  Port=5
  Arresting2 : Inport  Port=6
  Arresting3 : Inport  Port=7
  Arresting4 : Inport  Port=8
  C1 : Constant
  C2 : Constant
  C3 : Constant  Value=-1
  LTZone : $bdroot/Neuron Elements/LTZone  NM=1  FB=1.7  IT=0.005  T=0.1
  Simple Membrane{,1..3} (4 alike) : $bdroot/Neuron Elements/Simple Membrane  ACm=1e-9  ARm=1e7  ECm=1e-9  ERm=1e7  ARFm=1e8  ERFm=1e8
  Sum12 : Sum  InputSameDT=on  SaturateOnIntegerOverflow=on  OutDataTypeStr=Inherit: Same as first input
  Sum7 : Sum  InputSameDT=on  SaturateOnIntegerOverflow=on  OutDataTypeStr=Inherit: Same as first input
  Synapse{,1..7} (8 alike) : $bdroot/Neuron Elements/Synapse  SecretionTC=0.001  DecompositionTC=0.01  UseKsi=on  ksi=2  gamma=1e8
  Out : Outport  VectorParamsAs1DForOutWhenUnconnected=off
  Visual : Outport  Port=2  VectorParamsAs1DForOutWhenUnconnected=off
  Potential : Outport  Port=3  VectorParamsAs1DForOutWhenUnconnected=off
  wires:
  Synapse7/1 -> Simple Membrane/5
  Arresting4/1 -> Synapse7/1
  Synapse6/1 -> Simple Membrane1/5
  Arresting3/1 -> Synapse6/1
  Synapse5/1 -> Simple Membrane2/5
  Arresting2/1 -> Synapse5/1
  Stimulate4/1 -> Synapse4/1
  Synapse4/1 -> Simple Membrane/1
  Stimulate3/1 -> Synapse3/1
  Synapse3/1 -> Simple Membrane1/1
  Stimulate2/1 -> Synapse2/1
  Synapse2/1 -> Simple Membrane2/1
  Synapse/1 -> Simple Membrane3/1
  C2/1 -> Simple Membrane3/2
  C3/1 -> Simple Membrane3/4
  Synapse1/1 -> Simple Membrane3/5
  Simple Membrane3/2 -> Simple Membrane2/4
  Simple Membrane3/1 -> Simple Membrane2/2
  Simple Membrane2/2 -> Simple Membrane1/4
  Simple Membrane2/1 -> Simple Membrane1/2
  LTZone/2 -> Visual/1
  LTZone/3 -> Out/1
  C1/1 -> LTZone/2
  Stimulate1/1 -> Synapse/1
  Arresting1/1 -> Synapse1/1
  Simple Membrane1/1 -> Simple Membrane/2, Sum12/1
  Simple Membrane1/2 -> Simple Membrane/4, Sum12/2
  Sum7/1 -> LTZone/1, Potential/1
  LTZone/1 -> Simple Membrane/3
  Simple Membrane/1 -> Sum7/1
  Simple Membrane/2 -> Sum7/2

== system NeuroModelerLibrary/Dendrites Cells/Long Dendite Cell ModGen(FBC) ==
  Stimulate1 : Inport
  Stimulate2 : Inport  Port=2
  Stimulate3 : Inport  Port=3
  Stimulate4 : Inport  Port=4
  Arresting1 : Inport  Port=5
  Arresting2 : Inport  Port=6
  Arresting3 : Inport  Port=7
  Arresting4 : Inport  Port=8
  C1 : Constant
  C2 : Constant
  C3 : Constant  Value=-1
  LTZone : $bdroot/Neuron Elements/LTZone  NM=1  FB=2  IT=0.005  T=0.001
  Simple Membrane{,1..3} (4 alike) : $bdroot/Neuron Elements/Simple Membrane  ACm=1e-9  ARm=1e7  ECm=1e-9  ERm=1e7  ARFm=1e8  ERFm=1e8
  Sum12 : Sum  InputSameDT=on  SaturateOnIntegerOverflow=on  OutDataTypeStr=Inherit: Same as first input
  Sum7 : Sum  InputSameDT=on  SaturateOnIntegerOverflow=on  OutDataTypeStr=Inherit: Same as first input
  Synapse{,1..7} (8 alike) : $bdroot/Neuron Elements/Synapse  SecretionTC=0.001  DecompositionTC=0.01  UseKsi=on  ksi=1  gamma=1e8
  Out : Outport  VectorParamsAs1DForOutWhenUnconnected=off
  Visual : Outport  Port=2  VectorParamsAs1DForOutWhenUnconnected=off
  Potential : Outport  Port=3  VectorParamsAs1DForOutWhenUnconnected=off
  wires:
  Synapse/1 -> Simple Membrane3/1
  Synapse3/1 -> Simple Membrane1/1
  Simple Membrane/2 -> Sum7/2
  Simple Membrane/1 -> Sum7/1
  LTZone/1 -> Simple Membrane/3
  Sum7/1 -> Potential/1, LTZone/1
  Simple Membrane1/2 -> Sum12/2, Simple Membrane/4
  Simple Membrane1/1 -> Sum12/1, Simple Membrane/2
  Arresting1/1 -> Synapse1/1
  Stimulate1/1 -> Synapse/1
  C1/1 -> LTZone/2
  LTZone/3 -> Out/1
  LTZone/2 -> Visual/1
  Simple Membrane2/1 -> Simple Membrane1/2
  Simple Membrane2/2 -> Simple Membrane1/4
  Simple Membrane3/1 -> Simple Membrane2/2
  Simple Membrane3/2 -> Simple Membrane2/4
  Synapse1/1 -> Simple Membrane3/5
  C3/1 -> Simple Membrane3/4
  C2/1 -> Simple Membrane3/2
  Synapse2/1 -> Simple Membrane2/1
  Stimulate2/1 -> Synapse2/1
  Stimulate3/1 -> Synapse3/1
  Synapse4/1 -> Simple Membrane/1
  Stimulate4/1 -> Synapse4/1
  Arresting2/1 -> Synapse5/1
  Synapse5/1 -> Simple Membrane2/5
  Arresting3/1 -> Synapse6/1
  Synapse6/1 -> Simple Membrane1/5
  Arresting4/1 -> Synapse7/1
  Synapse7/1 -> Simple Membrane/5

== system NeuroModelerLibrary/Dendrites Cells/Long Dendite Cell ModGenSyn ==
  Stimulate1 : Inport
  Stimulate2 : Inport  Port=2
  Stimulate3 : Inport  Port=3
  Stimulate4 : Inport  Port=4
  Arresting1 : Inport  Port=5
  Arresting2 : Inport  Port=6
  Arresting3 : Inport  Port=7
  Arresting4 : Inport  Port=8
  C1 : Constant
  C2 : Constant
  C3 : Constant  Value=-1
  LTZone : $bdroot/Neuron Elements/LTZone  NM=1  FB=2  IT=0.005  T=0.1
  Simple Membrane{,1..3} (4 alike) : $bdroot/Neuron Elements/Simple Membrane  ACm=1e-9  ARm=1e7  ECm=1e-9  ERm=1e7  ARFm=1e8  ERFm=1e8
  Sum12 : Sum  InputSameDT=on  SaturateOnIntegerOverflow=on  OutDataTypeStr=Inherit: Same as first input
  Sum7 : Sum  InputSameDT=on  SaturateOnIntegerOverflow=on  OutDataTypeStr=Inherit: Same as first input
  Synapse{,1..7} (8 alike) : $bdroot/Neuron Elements/Synapse  SecretionTC=0.001  DecompositionTC=0.01  UseKsi=on  ksi=1  gamma=1e8
  Out : Outport
  Visual : Outport  Port=2
  Potential : Outport  Port=3
  wires:
  Simple Membrane/2 -> Sum7/2
  Simple Membrane/1 -> Sum7/1
  LTZone/1 -> Simple Membrane/3
  Sum7/1 -> Potential/1, LTZone/1
  Simple Membrane1/2 -> Sum12/2, Simple Membrane/4
  Simple Membrane1/1 -> Sum12/1, Simple Membrane/2
  Arresting1/1 -> Synapse1/1
  Stimulate1/1 -> Synapse/1
  C1/1 -> LTZone/2
  LTZone/3 -> Out/1
  LTZone/2 -> Visual/1
  Simple Membrane2/1 -> Simple Membrane1/2
  Simple Membrane2/2 -> Simple Membrane1/4
  Simple Membrane3/1 -> Simple Membrane2/2
  Simple Membrane3/2 -> Simple Membrane2/4
  Synapse1/1 -> Simple Membrane3/5
  C3/1 -> Simple Membrane3/4
  C2/1 -> Simple Membrane3/2
  Synapse/1 -> Simple Membrane3/1
  Synapse2/1 -> Simple Membrane2/1
  Stimulate2/1 -> Synapse2/1
  Synapse3/1 -> Simple Membrane1/1
  Stimulate3/1 -> Synapse3/1
  Synapse4/1 -> Simple Membrane/1
  Stimulate4/1 -> Synapse4/1
  Arresting2/1 -> Synapse5/1
  Synapse5/1 -> Simple Membrane2/5
  Arresting3/1 -> Synapse6/1
  Synapse6/1 -> Simple Membrane1/5
  Arresting4/1 -> Synapse7/1
  Synapse7/1 -> Simple Membrane/5

== system NeuroModelerLibrary/Memory Modules/Time-Memory Element ==
  Top-Level  Activate : Inport
  Prev Elem Activate : Inport  Port=2
  Bottom-Level  Deactivate : Inport  Port=3
  Size4 Cell : $bdroot/Sized Cells/Size4 Cell
  Size4 Cell1 : $bdroot/Sized Cells/Size4 Cell
  Size4 Cell2 : $bdroot/Sized Cells/Size4 Cell
  Bottom-Level  Control Output : Outport  VectorParamsAs1DForOutWhenUnconnected=off
  Next Elem  Activate : Outport  Port=2  VectorParamsAs1DForOutWhenUnconnected=off
  wires:
  Size4 Cell1/1 -> Size4 Cell/3, Size4 Cell/5
  Size4 Cell2/1 -> Next Elem  Activate/1, Size4 Cell/6, Size4 Cell1/5
  Top-Level  Activate/1 -> Size4 Cell/1
  Size4 Cell/1 -> Bottom-Level  Control Output/1, Size4 Cell1/1
  Prev Elem Activate/1 -> Size4 Cell/2
  Bottom-Level  Deactivate/1 -> Size4 Cell2/4

== system NeuroModelerLibrary/Memory Modules/Time-Memory PI Element ==
  Top-Level  Activate : Inport
  Prev Elem Activate : Inport  Port=2
  Bottom-Level  Deactivate : Inport  Port=3
  N1 : Subsystem  AncestorBlock=NeuroModelerLibrary/Sized Cells/Size4 Cell
  N2 : $bdroot/Sized Cells/Size4 Cell
  Bottom-Level  Control Output : Outport  VectorParamsAs1DForOutWhenUnconnected=off
  wires:
  N2/1 -> N1/3(Stimulate3)
  Bottom-Level  Deactivate/1 -> N2/5, N2/7, N1/7(Arresting3), N1/5(Arresting1)
  N1/1(Out) -> Bottom-Level  Control Output/1, N2/3
  Prev Elem Activate/1 -> N1/9(Arresting5), N1/8(Arresting4), N1/1(Stimulate1)
  Top-Level  Activate/1 -> N1/2(Stimulate2)

== system NeuroModelerLibrary/Multistate Cells/Multistate Membrane Cell ==
  Stimulate : Inport
  Arresting : Inport  Port=2
  C1 : Constant
  C2 : Constant
  C3 : Constant  Value=-1
  LTZone : $bdroot/Neuron Elements/LTZone  NM=1  FB=1.7  IT=0.005  T=0.001
  Multistate Membrane : $bdroot/Neuron Elements/Multistate Membrane  SystemSampleTime=-1  VariantActivationTime=update diagram  Latency=0  AutoFrameSizeCalculation=off
  Simple Membrane : $bdroot/Neuron Elements/Simple Membrane  ACm=1e-9  ARm=1e7  ECm=1e-9  ERm=1e7  ARFm=1e8  ERFm=1e8
  Sum12 : Sum  InputSameDT=on  SaturateOnIntegerOverflow=on  OutDataTypeStr=Inherit: Same as first input
  Sum7 : Sum  InputSameDT=on  SaturateOnIntegerOverflow=on  OutDataTypeStr=Inherit: Same as first input
  Synapse : $bdroot/Neuron Elements/Synapse  SecretionTC=0.001  DecompositionTC=0.01  UseKsi=on  ksi=2  gamma=1e8
  Synapse1 : $bdroot/Neuron Elements/Synapse  SecretionTC=0.001  DecompositionTC=0.01  UseKsi=on  ksi=2  gamma=1e8
  Out : Outport  VectorParamsAs1DForOutWhenUnconnected=off
  Visual : Outport  Port=2  VectorParamsAs1DForOutWhenUnconnected=off
  Potential : Outport  Port=3  VectorParamsAs1DForOutWhenUnconnected=off
  wires:
  Simple Membrane/2 -> Sum7/2
  Simple Membrane/1 -> Sum7/1
  Synapse1/1 -> Multistate Membrane/5
  Synapse/1 -> Multistate Membrane/1
  C3/1 -> Multistate Membrane/4
  C2/1 -> Multistate Membrane/2
  LTZone/1 -> Simple Membrane/3
  Sum7/1 -> LTZone/1
  Multistate Membrane/2 -> Sum12/2, Simple Membrane/4
  Multistate Membrane/1 -> Sum12/1, Simple Membrane/2
  Arresting/1 -> Synapse1/1
  Stimulate/1 -> Synapse/1
  C1/1 -> LTZone/2
  LTZone/3 -> Out/1
  LTZone/2 -> Visual/1
  Sum12/1 -> Potential/1

== system NeuroModelerLibrary/Neuron Elements/CSNM Compartment ==
  Excitatory Synapse : Inport
  Excitatory input : Inport  Port=2
  Feedback : Inport  Port=3
  Arresting input : Inport  Port=4
  Arresting Synapse : Inport  Port=5
  ACm : Constant  Value=ACm
  ARm : Constant  Value=ARm
  ARm1 : Constant  Value=ARFm
  ECm : Constant  Value=ECm
  ERm : Constant  Value=ERm
  ERm1 : Constant  Value=ERFm
  Gain1 : Gain  Gain=sign
  Gain11 : Gain  Gain=1/U0
  Ion System : $bdroot/Neuron Elements/Ion System  SystemSampleTime=-1  VariantActivationTime=update diagram  Latency=0  AutoFrameSizeCalculation=off
  Ion System1 : $bdroot/Neuron Elements/Ion System  SystemSampleTime=-1  VariantActivationTime=update diagram  Latency=0  AutoFrameSizeCalculation=off
  Excitatory Out : Outport  VectorParamsAs1DForOutWhenUnconnected=off
  Arresting Out : Outport  Port=2  VectorParamsAs1DForOutWhenUnconnected=off
  wires:
  Ion System1/1 -> Excitatory Out/1
  ERm1/1 -> Ion System1/6
  Ion System/1 -> Arresting Out/1
  ACm/1 -> Ion System/4
  ARm/1 -> Ion System/3
  ECm/1 -> Ion System1/4
  ERm/1 -> Ion System1/3
  Excitatory Synapse/1 -> Gain11/1
  Arresting Synapse/1 -> Ion System1/1
  Excitatory input/1 -> Ion System1/2
  ARm1/1 -> Ion System/6
  Feedback/1 -> Ion System1/5, Ion System/5
  Arresting input/1 -> Ion System/2
  Gain11/1 -> Gain1/1  "g"
  Gain1/1 -> Ion System/1  "g"

== system NeuroModelerLibrary/Neuron Elements/CSNM LTZone ==
  Potential : Inport
  E : Inport  Port=2
  C5 : Constant  Value=0
  FB : Gain  Gain=FB  OutDataTypeStr=Inherit: Same as input  ParamDataTypeStr=Inherit: Same as input
  Inputs : Gain  Gain=1/NM  OutDataTypeStr=Inherit: Same as input  ParamDataTypeStr=Inherit: Same as input
  Relay : Relay  OnSwitchValue=T  OffSwitchValue=switchOff
  S2 : Switch  Threshold=1  SaturateOnIntegerOverflow=on  InputSameDT=on
  S3 : Switch  Threshold=1  SaturateOnIntegerOverflow=on  InputSameDT=on
  Out : Outport  InitialOutput=0  VectorParamsAs1DForOutWhenUnconnected=off
  OutPotential : Outport  Port=2  InitialOutput=0  VectorParamsAs1DForOutWhenUnconnected=off
  Feedback : Outport  Port=3  InitialOutput=0  VectorParamsAs1DForOutWhenUnconnected=off
  Visual : Outport  Port=4  InitialOutput=0  VectorParamsAs1DForOutWhenUnconnected=off
  wires:
  FB/1 -> Feedback/1
  Potential/1 -> Inputs/1
  C5/1 -> S2/3
  E/1 -> S2/1, S3/1
  S2/1 -> Out/1, FB/1
  Relay/1 -> S2/2, S3/2
  S3/1 -> Visual/1
  Inputs/1 -> OutPotential/1, Relay/1

== system NeuroModelerLibrary/Neuron Elements/CSNM Synapse ==
  pulse input : Inport
  Constant : Constant
  Constant1 : Constant  Value=0
  Constant2 : Constant  Value=UseKsi
  Constant3 : Constant  Value=-1
  Constant4 : Constant  Value=DecompositionTC
  Constant5 : Constant  Value=SecretionTC
  Constant6 : Constant  Value=sign
  Fcn : Fcn  Expr=u*u*ksi
  Gain : Gain  Gain=4*ksi/Rs  SaturateOnIntegerOverflow=on  OutDataTypeStr=Inherit: Same as input  ParamDataTypeStr=Inherit: Same as input
  Gain1 : Gain  SaturateOnIntegerOverflow=on  OutDataTypeStr=Inherit: Same as input  ParamDataTypeStr=Inherit: Same as input
  Gain2 : Gain  Gain=1/Rs  SaturateOnIntegerOverflow=on  OutDataTypeStr=Inherit: Same as input  ParamDataTypeStr=Inherit: Same as input
  Gain4 : Gain  Gain=Weight
  Gain9 : Gain  Gain=U0
  Inertial Link : $bdroot/Support/Inertial Link  SystemSampleTime=-1  VariantActivationTime=update diagram  Latency=0  AutoFrameSizeCalculation=off
  Product : Product
  Sum : Sum  Inputs=+-  SaturateOnIntegerOverflow=on
  Switch : Switch  Threshold=1
  Switch1 : Switch
  Switch2 : Switch  Threshold=1
  Switch3 : Switch  Threshold=1
  i_syn : Outport  VectorParamsAs1DForOutWhenUnconnected=off
  wires:
  Gain2/1 -> Switch3/3
  Constant2/1 -> Switch3/2
  Switch3/1 -> Switch1/2, Switch1/1
  Gain/1 -> Switch3/1
  Switch1/1 -> Gain9/1
  Gain1/1 -> Inertial Link/1
  Constant1/1 -> Switch1/3
  Switch2/1 -> Inertial Link/2
  Constant5/1 -> Switch2/1
  Constant4/1 -> Switch2/3
  Inertial Link/1 -> Sum/1, Fcn/1, Gain2/1
  Sum/1 -> Gain/1
  pulse input/1 -> Gain1/1, Switch2/2
  Fcn/1 -> Sum/2
  Gain9/1 -> Product/2
  Product/1 -> Gain4/1
  Gain4/1 -> i_syn/1
  Constant6/1 -> Switch/2
  Constant/1 -> Switch/1
  Constant3/1 -> Switch/3
  Switch/1 -> Product/1

== system NeuroModelerLibrary/Neuron Elements/CSNM Synapse-D ==
  In1 : Inport
  Clock1 : Clock
  Constant : Constant
  Constant1 : Constant  Value=0
  Constant2 : Constant  Value=UseKsi
  Constant3 : Constant  Value=-1
  Constant4 : Constant  Value=DecompositionTC
  Constant5 : Constant  Value=SecretionTC
  Constant6 : Constant  Value=sign
  Constant7 : Constant  Value=0
  Constant8 : Constant
  Fcn : Fcn  Expr=u*u*ksi
  Gain : Gain  Gain=4*ksi/Rs  SaturateOnIntegerOverflow=on  OutDataTypeStr=Inherit: Same as input  ParamDataTypeStr=Inherit: Same as input
  Gain1 : Gain  SaturateOnIntegerOverflow=on  OutDataTypeStr=Inherit: Same as input  ParamDataTypeStr=Inherit: Same as input
  Gain2 : Gain  Gain=1/Rs  SaturateOnIntegerOverflow=on  OutDataTypeStr=Inherit: Same as input  ParamDataTypeStr=Inherit: Same as input
  Gain4 : Gain  Gain=Weight
  Gain9 : Gain  Gain=U0
  Inertial Link : $bdroot/Support/Inertial Link  SystemSampleTime=-1  VariantActivationTime=update diagram  Latency=0  AutoFrameSizeCalculation=off
  Product : Product
  Sum : Sum  Inputs=+-  SaturateOnIntegerOverflow=on
  Sum1 : Sum  Inputs=-+|
  Switch : Switch  Threshold=1
  Switch1 : Switch
  Switch2 : Switch  Threshold=1
  Switch3 : Switch  Threshold=1
  Switch4 : Switch  Threshold=0.001  SaturateOnIntegerOverflow=on  InputSameDT=on
  Triggered Subsystem : Subsystem  TreatAsAtomicUnit=on
  Out1 : Outport  VectorParamsAs1DForOutWhenUnconnected=off
  wires:
  Gain2/1 -> Switch3/3
  Constant2/1 -> Switch3/2
  Switch3/1 -> Switch1/2, Switch1/1
  Gain/1 -> Switch3/1
  Switch1/1 -> Gain9/1
  Gain1/1 -> Inertial Link/1
  Constant1/1 -> Switch1/3
  Switch2/1 -> Inertial Link/2
  Constant5/1 -> Switch2/1
  Constant4/1 -> Switch2/3
  Inertial Link/1 -> Sum/1, Fcn/1, Gain2/1
  Sum/1 -> Gain/1
  Fcn/1 -> Sum/2
  Gain9/1 -> Product/2
  Product/1 -> Gain4/1
  Gain4/1 -> Out1/1
  Switch/1 -> Product/1
  Constant6/1 -> Switch/2
  Constant/1 -> Switch/1
  Constant3/1 -> Switch/3
  Triggered Subsystem/1(Out1) -> Sum1/1
  Sum1/1 -> Switch4/2
  Constant8/1 -> Switch4/3
  Clock1/1 -> Sum1/2, Triggered Subsystem/1(In1)
  Constant7/1 -> Switch4/1
  In1/1 -> Triggered Subsystem/Trigger
  Switch4/1 -> Switch2/2, Gain1/1

== system NeuroModelerLibrary/Neuron Elements/ContLTZone ==
  In1 : Inport
  Compare To Zero2 : simulink/Logic and Bit Operations/Compare To Zero  relop=>=  OutDataTypeStr=uint8  ZeroCross=off
  Product2 : Product  RndMeth=Zero
  Sign2 : Signum
  tansig : neural/Transfer Functions/tansig
  Out1 : Outport  VectorParamsAs1DForOutWhenUnconnected=off
  wires:
  Product2/1 -> Out1/1
  In1/1 -> tansig/1
  tansig/1 -> Product2/1, Sign2/1
  Compare To Zero2/1 -> Product2/2
  Sign2/1 -> Compare To Zero2/1
